simulink subsystem "Kinematics_313"  (R2022b)
settings: Solver=VariableStepAuto  StartTime=0.0  StopTime=10.0  RelTol=1e-3
undefined symbols (not defined in the file or in its folder): E0
settings Model: Creator=brent  LastModifiedBy=brent

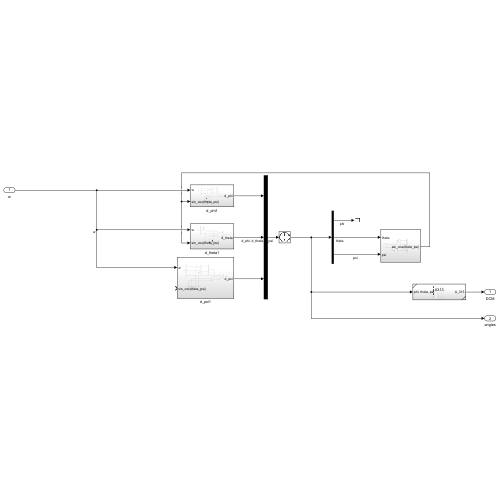
[thumbnail: Simulink's stored preview of the top-level diagram]
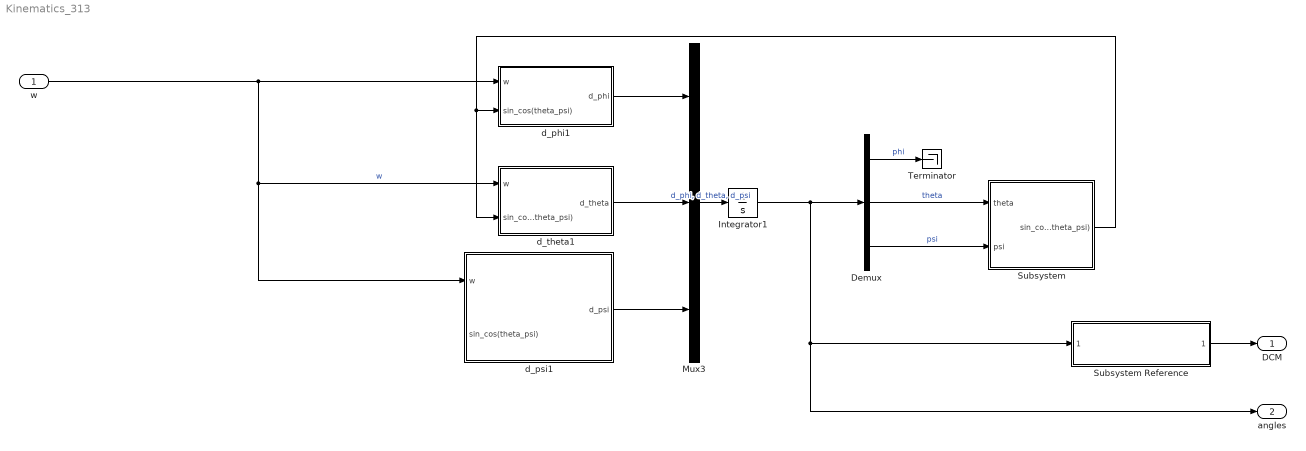
== system Kinematics_313 ==
  w : Inport
  Demux : Demux  Outputs=3
  Integrator1 : Integrator  InitialCondition=E0  WrapState=on
  Mux3 : Mux  Inputs=3
  Subsystem : Subsystem
  Subsystem Reference : Subsystem  ReferencedSubsystem=A313
  Terminator : Terminator
  d_phi1 : Subsystem
  d_psi1 : Subsystem
  d_theta1 : Subsystem
  DCM : Outport
  angles : Outport  Port=2
  wires:
  w/1 -> d_psi1/1(w), d_theta1/1(w), d_phi1/1(w)  "w"
  Integrator1/1 -> Subsystem Reference/1, angles/1, Demux/1
  Demux/3 -> Subsystem/2(psi)  "psi"
  Demux/1 -> Terminator/1  "phi"
  d_psi1/1(d_psi) -> Mux3/3
  d_theta1/1(d_theta) -> Mux3/2
  d_phi1/1(d_phi) -> Mux3/1
  Subsystem/1(sin_cos(theta_psi)) -> d_theta1/2(sin_cos(theta_psi)), d_phi1/2(sin_cos(theta_psi))
  Demux/2 -> Subsystem/1(theta)  "theta"
  Mux3/1 -> Integrator1/1  "d_phi, d_theta, d_psi"
  Subsystem Reference/1 -> DCM/1

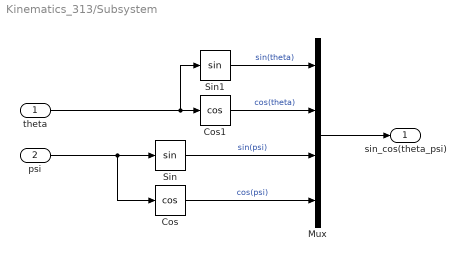
== system Kinematics_313/Subsystem ==
  theta : Inport
  psi : Inport  Port=2
  Cos : Trigonometry  Operator=cos
  Cos1 : Trigonometry  Operator=cos
  Mux : Mux
  Sin : Trigonometry
  Sin1 : Trigonometry
  sin_cos(theta_psi) : Outport
  wires:
  theta/1 -> Sin1/1, Cos1/1
  psi/1 -> Cos/1, Sin/1
  Sin1/1 -> Mux/1  "sin(theta)"
  Cos1/1 -> Mux/2  "cos(theta)"
  Sin/1 -> Mux/3  "sin(psi)"
  Cos/1 -> Mux/4  "cos(psi)"
  Mux/1 -> sin_cos(theta_psi)/1

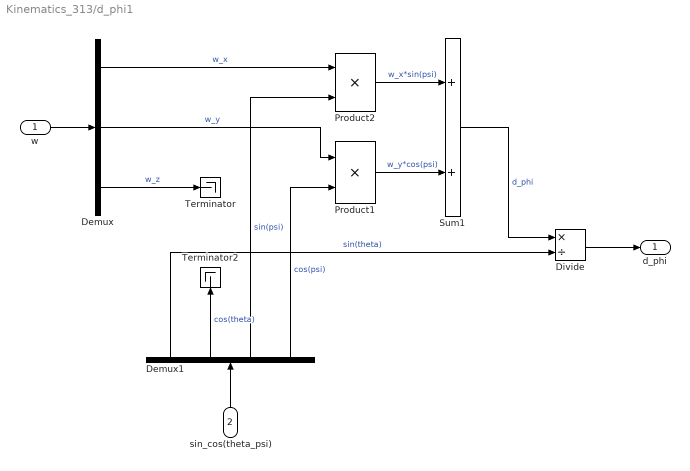
== system Kinematics_313/d_phi1 ==
  w : Inport
  sin_cos(theta_psi) : Inport  Port=2
  Demux : Demux  Outputs=3
  Demux1 : Demux
  Divide : Product  Inputs=*/
  Product1 : Product
  Product2 : Product
  Sum1 : Sum
  Terminator : Terminator
  Terminator2 : Terminator
  d_phi : Outport
  wires:
  Demux1/3 -> Product2/2  "sin(psi)"
  Demux/2 -> Product1/1  "w_y"
  Sum1/1 -> Divide/1  "d_phi"
  Product1/1 -> Sum1/2  "w_y*cos(psi)"
  Product2/1 -> Sum1/1  "w_x*sin(psi)"
  w/1 -> Demux/1
  Demux/3 -> Terminator/1  "w_z"
  Demux/1 -> Product2/1  "w_x"
  Demux1/2 -> Terminator2/1  "cos(theta)"
  Demux1/1 -> Divide/2  "sin(theta)"
  sin_cos(theta_psi)/1 -> Demux1/1
  Demux1/4 -> Product1/2  "cos(psi)"
  Divide/1 -> d_phi/1

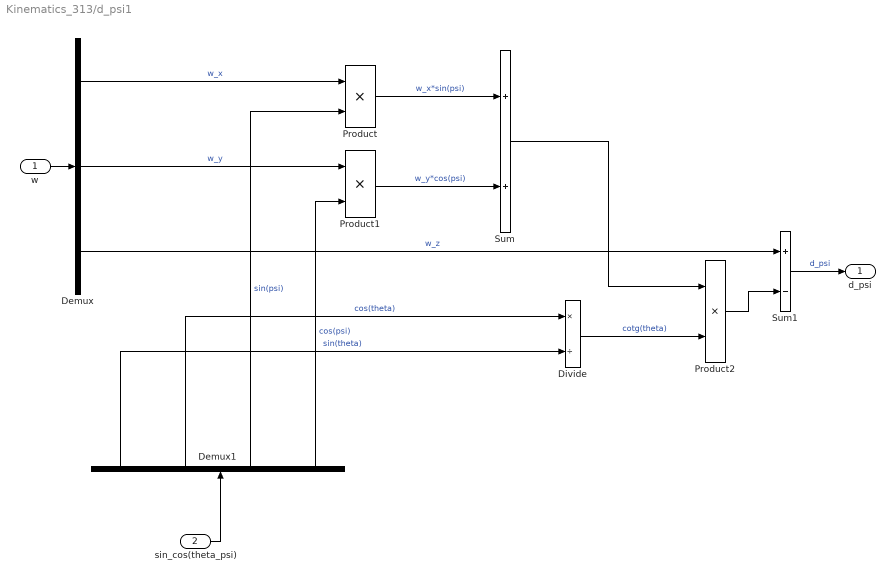
== system Kinematics_313/d_psi1 ==
  w : Inport
  sin_cos(theta_psi) : Inport  Port=2
  Demux : Demux  Outputs=3
  Demux1 : Demux
  Divide : Product  Inputs=*/
  Product : Product
  Product1 : Product
  Product2 : Product
  Sum : Sum
  Sum1 : Sum  Inputs=+-
  d_psi : Outport
  wires:
  Sum/1 -> Product2/1
  Divide/1 -> Product2/2  "cotg(theta)"
  Demux/3 -> Sum1/1  "w_z"
  Product1/1 -> Sum/2  "w_y*cos(psi)"
  Product2/1 -> Sum1/2
  Sum1/1 -> d_psi/1  "d_psi"
  Product/1 -> Sum/1  "w_x*sin(psi)"
  w/1 -> Demux/1
  Demux/1 -> Product/1  "w_x"
  Demux/2 -> Product1/1  "w_y"
  Demux1/2 -> Divide/1  "cos(theta)"
  sin_cos(theta_psi)/1 -> Demux1/1
  Demux1/1 -> Divide/2  "sin(theta)"
  Demux1/3 -> Product/2  "sin(psi)"
  Demux1/4 -> Product1/2  "cos(psi)"

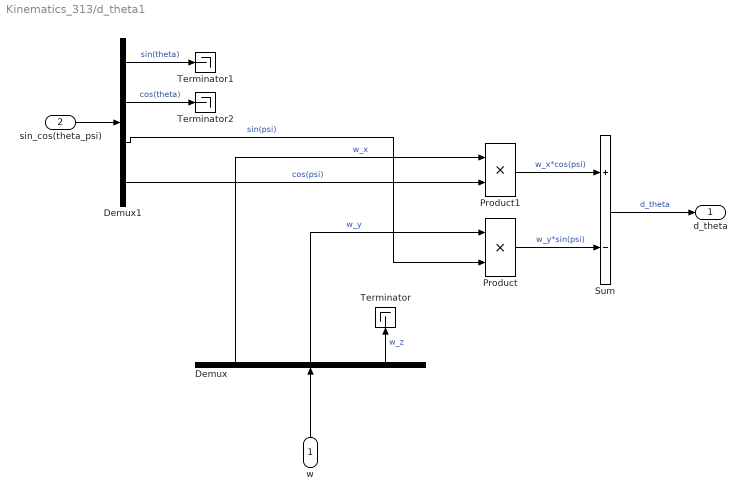
== system Kinematics_313/d_theta1 ==
  w : Inport
  sin_cos(theta_psi) : Inport  Port=2
  Demux : Demux  Outputs=3
  Demux1 : Demux
  Product : Product
  Product1 : Product
  Sum : Sum  Inputs=+-
  Terminator : Terminator
  Terminator1 : Terminator
  Terminator2 : Terminator
  d_theta : Outport
  wires:
  Demux/2 -> Product/1  "w_y"
  Demux1/3 -> Product/2  "sin(psi)"
  Product/1 -> Sum/2  "w_y*sin(psi)"
  Demux/1 -> Product1/1  "w_x"
  Sum/1 -> d_theta/1  "d_theta"
  Product1/1 -> Sum/1  "w_x*cos(psi)"
  w/1 -> Demux/1
  Demux/3 -> Terminator/1  "w_z"
  Demux1/2 -> Terminator2/1  "cos(theta)"
  Demux1/4 -> Product1/2  "cos(psi)"
  sin_cos(theta_psi)/1 -> Demux1/1
  Demux1/1 -> Terminator1/1  "sin(theta)"
